simulink model "Inverter_Arch"  (R2022b)
settings: Solver=FixedStepDiscrete  StartTime=0.0  StopTime=10.0  RelTol=1e-3
undefined symbols (not defined in the file): Vdc
settings Model: Creator=MAAM  LastModifiedBy=MAAM

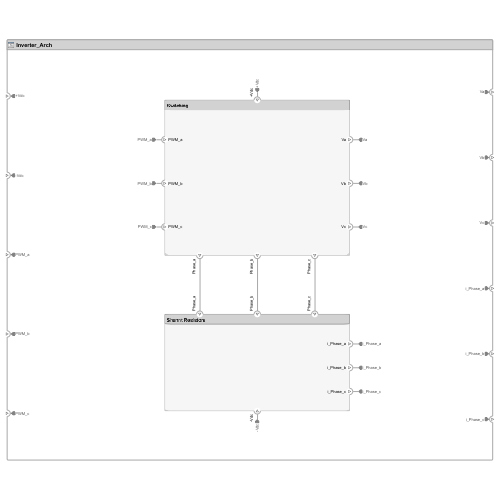
[thumbnail: Simulink's stored preview of the top-level diagram]
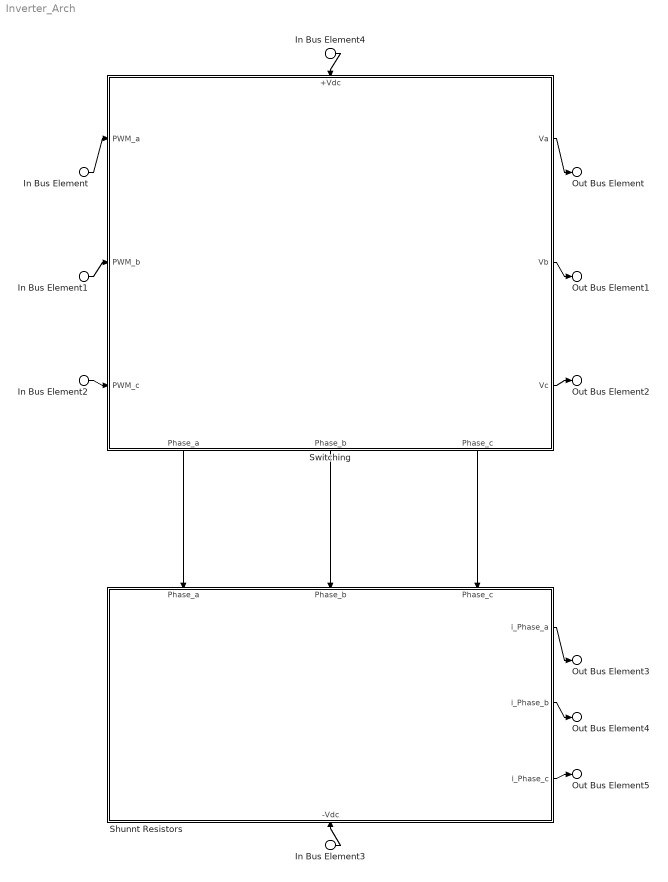
== system Inverter_Arch ==
  In Bus Element4 : Inport  PortName=+Vdc
  In Bus Element3 : Inport  Port=2  PortName=-Vdc
  In Bus Element : Inport  Port=3  PortName=PWM_a
  In Bus Element1 : Inport  Port=4  PortName=PWM_b
  In Bus Element2 : Inport  Port=5  PortName=PWM_c
  Shunnt Resistors : Subsystem
      settings: PortSchema="{\"entries\":[{\"content\":{\"headerSize\":26,\"margin\":15,\"minimumSpacing\":25,\"sides\":[{\"content\":{\"connectorIds\":[]},\"type\":\"ConnectorPlacement.EquallySpacedRectSide\",\"uuid\":\"ecb73a61-b18a-4e6f-9a16-a7412467d3dc\"},{\"content\":{\"connectorIds\":[\"Out1\",\"Out2\",\"Out3\"],\"side\":\"RIGHT\"},\"type\":\"ConnectorPlacement.EquallySpacedRectSide\",\"uuid\":\"05d75da6-23d5-4864-9569-f2b0c11a82bb\"},{\"content\":{\"connectorIds\":[\"In2\",\"In3\",\"In4\"],\"side\":\"TOP\"},\"type\":\"ConnectorPlacement.EquallySpacedRectSide\",\"uuid\":\"f7c561b3-9491-4c59-9ccb-7eaec9c6a3d8\"},{\"content\":{\"connectorIds\":[\"In1\"],\"side\":\"BOTTOM\"},\"type\":\"ConnectorPlacement.EquallySpacedRectSide\",\"uuid\":\"cad1b61f-6a65-4191-8f08-cc00b6213deb\"}]},\"type\":\"ConnectorPlacement.EquallySpacedConnector\",\"uuid\":\"7fcac072-6609-4f2b-820d-d62cc0efbf31\"}],\"packageUris\":[\"http://schema.mathworks.com/mf0/Connector/R2020b\"],\"version\":\"1.0\"}"
  Switching : Subsystem
      settings: PortSchema="{\"entries\":[{\"content\":{\"headerSize\":26,\"margin\":15,\"minimumSpacing\":25,\"sides\":[{\"content\":{\"connectorIds\":[\"In2\",\"In3\",\"In4\"]},\"type\":\"ConnectorPlacement.EquallySpacedRectSide\",\"uuid\":\"ecb73a61-b18a-4e6f-9a16-a7412467d3dc\"},{\"content\":{\"connectorIds\":[\"Out4\",\"Out5\",\"Out6\"],\"side\":\"RIGHT\"},\"type\":\"ConnectorPlacement.EquallySpacedRectSide\",\"uuid\":\"05d75da6-23d5-4864-9569-f2b0c11a82bb\"},{\"content\":{\"connectorIds\":[\"In1\"],\"side\":\"TOP\"},\"type\":\"ConnectorPlacement.EquallySpacedRectSide\",\"uuid\":\"f7c561b3-9491-4c59-9ccb-7eaec9c6a3d8\"},{\"content\":{\"connectorIds\":[\"Out1\",\"Out2\",\"Out3\"],\"side\":\"BOTTOM\"},\"type\":\"ConnectorPlacement.EquallySpacedRectSide\",\"uuid\":\"baa5380d-922a-4783-9d38-c6d4e2ad9f9d\"}]},\"type\":\"ConnectorPlacement.EquallySpacedConnector\",\"uuid\":\"7fcac072-6609-4f2b-820d-d62cc0efbf31\"}],\"packageUris\":[\"http://schema.mathworks.com/mf0/Connector/R2020b\"],\"version\":\"1.0\"}"
  Out Bus Element : Outport  PortName=Va
  Out Bus Element1 : Outport  Port=2  PortName=Vb
  Out Bus Element2 : Outport  Port=3  PortName=Vc
  Out Bus Element3 : Outport  Port=4  PortName=i_Phase_a
  Out Bus Element4 : Outport  Port=5  PortName=i_Phase_b
  Out Bus Element5 : Outport  Port=6  PortName=i_Phase_c
  wires:
  In Bus Element/1 -> Switching/2(PWM_a)
  Switching/4(Va) -> Out Bus Element/1
  In Bus Element2/1 -> Switching/4(PWM_c)
  In Bus Element1/1 -> Switching/3(PWM_b)
  Switching/6(Vc) -> Out Bus Element2/1
  Switching/5(Vb) -> Out Bus Element1/1
  Switching/1(Phase_a) -> Shunnt Resistors/2(Phase_a)
  Switching/2(Phase_b) -> Shunnt Resistors/3(Phase_b)
  Switching/3(Phase_c) -> Shunnt Resistors/4(Phase_c)
  Shunnt Resistors/1(i_Phase_a) -> Out Bus Element3/1
  Shunnt Resistors/2(i_Phase_b) -> Out Bus Element4/1
  Shunnt Resistors/3(i_Phase_c) -> Out Bus Element5/1
  In Bus Element4/1 -> Switching/1(+Vdc)
  In Bus Element3/1 -> Shunnt Resistors/1(-Vdc)

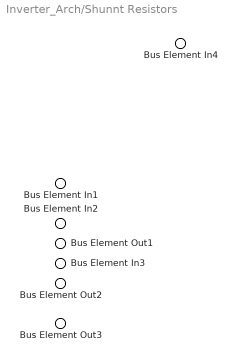
== system Inverter_Arch/Shunnt Resistors ==
  Bus Element In4 : Inport  PortName=-Vdc
  Bus Element In1 : Inport  Port=2  PortName=Phase_a
  Bus Element In2 : Inport  Port=3  PortName=Phase_b
  Bus Element In3 : Inport  Port=4  PortName=Phase_c
  Bus Element Out1 : Outport  PortName=i_Phase_a
  Bus Element Out2 : Outport  Port=2  PortName=i_Phase_b
  Bus Element Out3 : Outport  Port=3  PortName=i_Phase_c

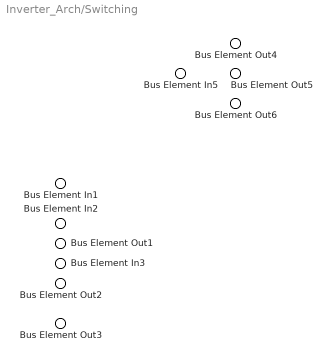
== system Inverter_Arch/Switching ==
  Bus Element In5 : Inport  PortName=+Vdc
  Bus Element In1 : Inport  Port=2  PortName=PWM_a
  Bus Element In2 : Inport  Port=3  PortName=PWM_b
  Bus Element In3 : Inport  Port=4  PortName=PWM_c
  Bus Element Out4 : Outport  PortName=Phase_a
  Bus Element Out5 : Outport  Port=2  PortName=Phase_b
  Bus Element Out6 : Outport  Port=3  PortName=Phase_c
  Bus Element Out1 : Outport  Port=4  PortName=Va
  Bus Element Out2 : Outport  Port=5  PortName=Vb
  Bus Element Out3 : Outport  Port=6  PortName=Vc
